simulink model "VCU_CS75_9_30"  (R2014a)
settings: Solver=FixedStepDiscrete  StartTime=0.0  StopTime=25  FixedStep=0.0005  RelTol=1e-3
undefined symbols (not defined in the file or in its folder): APAStatus_2D4, ecucoder_acal, I_SW01_L, LDW, ST_comd, TX2D4
libraries: simulink x881, ec5744lib x37
(part 29 of 30)

== system VCU_CS75_9_30/长安CS75底盘程序，20ms一次/BSW_Input/CAN1_Rx/SAS_108/ReceiveMessages/Subsystem/SAS_2 ==
  input : Inport
  Data Type Conversion : DataTypeConversion
  Demux : Demux  Outputs=8
  SAS_CRCCheck_Ad : Sum
  SAS_CRCCheck_Convert : DataTypeConversion  OutDataTypeStr=uint32
  SAS_CRCCheck_F : Gain
  SAS_CRCCheck_L : simulink/Logic and Bit Operations/Bitwise Operator  logicop=AND  UseBitMask=on  BitMask=255  BitMaskRealWorld=Stored Integer
  SAS_CRCCheck_O : Constant  Value=0  OutDataTypeStr=single
  SAS_CRCCheck_S : ArithShift
  SAS_CRCCheck_Sub : Subsystem
  SAS_CRCCheck_sat : Saturate  UpperLimit=255  LowerLimit=0
  SAS_CRCCheckcv : DataTypeConversion
  SAS_Calibrated_Ad : Sum
  SAS_Calibrated_Convert : DataTypeConversion  OutDataTypeStr=uint32
  SAS_Calibrated_F : Gain
  SAS_Calibrated_L : simulink/Logic and Bit Operations/Bitwise Operator  logicop=AND  UseBitMask=on  BitMask=32  BitMaskRealWorld=Stored Integer
  SAS_Calibrated_O : Constant  Value=0  OutDataTypeStr=single
  SAS_Calibrated_S : ArithShift  BitShiftNumber=5
  SAS_Calibrated_Sub : Subsystem
  SAS_Calibrated_sat : Saturate  UpperLimit=1  LowerLimit=0
  SAS_Calibratedcv : DataTypeConversion
  SAS_RollingCounter_Ad : Sum
  SAS_RollingCounter_Convert : DataTypeConversion  OutDataTypeStr=uint32
  SAS_RollingCounter_F : Gain
  SAS_RollingCounter_L : simulink/Logic and Bit Operations/Bitwise Operator  logicop=AND  UseBitMask=on  BitMask=15  BitMaskRealWorld=Stored Integer
  SAS_RollingCounter_O : Constant  Value=0  OutDataTypeStr=single
  SAS_RollingCounter_S : ArithShift
  SAS_RollingCounter_Sub : Subsystem
  SAS_RollingCounter_sat : Saturate  UpperLimit=15  LowerLimit=0
  SAS_RollingCountercv : DataTypeConversion
  SAS_SASFailure_Ad : Sum
  SAS_SASFailure_Convert : DataTypeConversion  OutDataTypeStr=uint32
  SAS_SASFailure_F : Gain
  SAS_SASFailure_L : simulink/Logic and Bit Operations/Bitwise Operator  logicop=AND  UseBitMask=on  BitMask=64  BitMaskRealWorld=Stored Integer
  SAS_SASFailure_O : Constant  Value=0  OutDataTypeStr=single
  SAS_SASFailure_S : ArithShift  BitShiftNumber=6
  SAS_SASFailure_Sub : Subsystem
  SAS_SASFailure_sat : Saturate  UpperLimit=1  LowerLimit=0
  SAS_SASFailurecv : DataTypeConversion
  SAS_SteeringAngleCS : ArithShift  BitShiftNumber=-16
  SAS_SteeringAngleCS1 : ArithShift  BitShiftNumber=-15
  SAS_SteeringAngleConS : Constant  OutDataTypeStr=single
  SAS_SteeringAngleMinus : UnaryMinus
  SAS_SteeringAngleROP : RelationalOperator  OutDataTypeStr=boolean
  SAS_SteeringAngleSW : Switch  Criteria=u2 ~= 0
  SAS_SteeringAngleSpeed_Ad : Sum
  SAS_SteeringAngleSpeed_Convert : DataTypeConversion  OutDataTypeStr=uint32
  SAS_SteeringAngleSpeed_F : Gain  Gain=4
  SAS_SteeringAngleSpeed_L : simulink/Logic and Bit Operations/Bitwise Operator  logicop=AND  UseBitMask=on  BitMask=255  BitMaskRealWorld=Stored Integer
  SAS_SteeringAngleSpeed_O : Constant  Value=0  OutDataTypeStr=single
  SAS_SteeringAngleSpeed_S : ArithShift
  SAS_SteeringAngleSpeed_Sub : Subsystem
  SAS_SteeringAngleSpeed_sat : Saturate  UpperLimit=1020  LowerLimit=0
  SAS_SteeringAngleSpeedcv : DataTypeConversion
  SAS_SteeringAngleValid_Ad : Sum
  SAS_SteeringAngleValid_Convert : DataTypeConversion  OutDataTypeStr=uint32
  SAS_SteeringAngleValid_F : Gain
  SAS_SteeringAngleValid_L : simulink/Logic and Bit Operations/Bitwise Operator  logicop=AND  UseBitMask=on  BitMask=128  BitMaskRealWorld=Stored Integer
  SAS_SteeringAngleValid_O : Constant  Value=0  OutDataTypeStr=single
  SAS_SteeringAngleValid_S : ArithShift  BitShiftNumber=7
  SAS_SteeringAngleValid_Sub : Subsystem
  SAS_SteeringAngleValid_sat : Saturate  UpperLimit=1  LowerLimit=0
  SAS_SteeringAngleValidcv : DataTypeConversion
  SAS_SteeringAngle_Ad : Sum
  SAS_SteeringAngle_Convert : DataTypeConversion  OutDataTypeStr=uint32
  SAS_SteeringAngle_F : Gain  Gain=0.1
  SAS_SteeringAngle_L : simulink/Logic and Bit Operations/Bitwise Operator  logicop=AND  UseBitMask=on  BitMask=65535  BitMaskRealWorld=Stored Integer
  SAS_SteeringAngle_O : Constant  Value=0  OutDataTypeStr=single
  SAS_SteeringAngle_S : ArithShift
  SAS_SteeringAngle_Sub : Subsystem
  SAS_SteeringAngle_sat : Saturate  UpperLimit=780  LowerLimit=-780
  SAS_SteeringAnglecv : DataTypeConversion
  SAS_SteeringAngleinput1_Ad : Sum
  SAS_SteeringAngleinput1_C : Constant  Value=256
  SAS_SteeringAngleinput1_P : Product
  SAS_SteeringAnglesubcon : Sum  Inputs=+-
  SAS_SteeringAngle_Out : Outport
  SAS_SteeringAngleSpeed_Out : Outport  Port=2
  SAS_Calibrated_Out : Outport  Port=3
  SAS_SASFailure_Out : Outport  Port=4
  SAS_SteeringAngleValid_Out : Outport  Port=5
  SAS_RollingCounter_Out : Outport  Port=6
  SAS_CRCCheck_Out : Outport  Port=7
  wires:
  SAS_SteeringAngle_F/1 -> SAS_SteeringAngle_Ad/1
  SAS_SteeringAngle_O/1 -> SAS_SteeringAngle_Ad/2
  SAS_SteeringAngle_Ad/1 -> SAS_SteeringAngle_sat/1
  SAS_SteeringAngle_sat/1 -> SAS_SteeringAngle_Out/1
  Demux/1 -> SAS_SteeringAngleinput1_P/1
  SAS_SteeringAngleinput1_C/1 -> SAS_SteeringAngleinput1_P/2
  SAS_SteeringAngleinput1_P/1 -> SAS_SteeringAngleinput1_Ad/1
  Demux/2 -> SAS_SteeringAngleinput1_Ad/2
  SAS_SteeringAngleinput1_Ad/1 -> SAS_SteeringAngle_Sub/1(In1)
  SAS_SteeringAngle_Sub/1(Out1) -> SAS_SteeringAngle_Convert/1
  SAS_SteeringAngle_Convert/1 -> SAS_SteeringAngle_L/1
  SAS_SteeringAngle_L/1 -> SAS_SteeringAngle_S/1
  SAS_SteeringAngle_S/1 -> SAS_SteeringAnglecv/1
  SAS_SteeringAnglecv/1 -> SAS_SteeringAngleROP/1, SAS_SteeringAnglesubcon/2, SAS_SteeringAngleSW/3
  SAS_SteeringAngleConS/1 -> SAS_SteeringAngleCS/1, SAS_SteeringAngleCS1/1
  SAS_SteeringAngleCS1/1 -> SAS_SteeringAngleROP/2
  SAS_SteeringAngleCS/1 -> SAS_SteeringAnglesubcon/1
  SAS_SteeringAnglesubcon/1 -> SAS_SteeringAngleMinus/1
  SAS_SteeringAngleMinus/1 -> SAS_SteeringAngleSW/1
  SAS_SteeringAngleSW/1 -> Data Type Conversion/1
  SAS_SteeringAngleROP/1 -> SAS_SteeringAngleSW/2
  SAS_SteeringAngleSpeed_F/1 -> SAS_SteeringAngleSpeed_Ad/1
  SAS_SteeringAngleSpeed_O/1 -> SAS_SteeringAngleSpeed_Ad/2
  SAS_SteeringAngleSpeed_Ad/1 -> SAS_SteeringAngleSpeed_sat/1
  SAS_SteeringAngleSpeed_sat/1 -> SAS_SteeringAngleSpeed_Out/1
  Demux/3 -> SAS_SteeringAngleSpeed_Sub/1(In1)
  SAS_SteeringAngleSpeed_Sub/1(Out1) -> SAS_SteeringAngleSpeed_Convert/1
  SAS_SteeringAngleSpeed_Convert/1 -> SAS_SteeringAngleSpeed_L/1
  SAS_SteeringAngleSpeed_L/1 -> SAS_SteeringAngleSpeed_S/1
  SAS_SteeringAngleSpeed_S/1 -> SAS_SteeringAngleSpeedcv/1
  SAS_SteeringAngleSpeedcv/1 -> SAS_SteeringAngleSpeed_F/1
  SAS_Calibrated_F/1 -> SAS_Calibrated_Ad/1
  SAS_Calibrated_O/1 -> SAS_Calibrated_Ad/2
  SAS_Calibrated_Ad/1 -> SAS_Calibrated_sat/1
  SAS_Calibrated_sat/1 -> SAS_Calibrated_Out/1
  Demux/4 -> SAS_Calibrated_Sub/1(In1), SAS_SASFailure_Sub/1(In1), SAS_SteeringAngleValid_Sub/1(In1)
  SAS_Calibrated_Sub/1(Out1) -> SAS_Calibrated_Convert/1
  SAS_Calibrated_Convert/1 -> SAS_Calibrated_L/1
  SAS_Calibrated_L/1 -> SAS_Calibrated_S/1
  SAS_Calibrated_S/1 -> SAS_Calibratedcv/1
  SAS_Calibratedcv/1 -> SAS_Calibrated_F/1
  SAS_SASFailure_F/1 -> SAS_SASFailure_Ad/1
  SAS_SASFailure_O/1 -> SAS_SASFailure_Ad/2
  SAS_SASFailure_Ad/1 -> SAS_SASFailure_sat/1
  SAS_SASFailure_sat/1 -> SAS_SASFailure_Out/1
  SAS_SASFailure_Sub/1(Out1) -> SAS_SASFailure_Convert/1
  SAS_SASFailure_Convert/1 -> SAS_SASFailure_L/1
  SAS_SASFailure_L/1 -> SAS_SASFailure_S/1
  SAS_SASFailure_S/1 -> SAS_SASFailurecv/1
  SAS_SASFailurecv/1 -> SAS_SASFailure_F/1
  SAS_SteeringAngleValid_F/1 -> SAS_SteeringAngleValid_Ad/1
  SAS_SteeringAngleValid_O/1 -> SAS_SteeringAngleValid_Ad/2
  SAS_SteeringAngleValid_Ad/1 -> SAS_SteeringAngleValid_sat/1
  SAS_SteeringAngleValid_sat/1 -> SAS_SteeringAngleValid_Out/1
  SAS_SteeringAngleValid_Sub/1(Out1) -> SAS_SteeringAngleValid_Convert/1
  SAS_SteeringAngleValid_Convert/1 -> SAS_SteeringAngleValid_L/1
  SAS_SteeringAngleValid_L/1 -> SAS_SteeringAngleValid_S/1
  SAS_SteeringAngleValid_S/1 -> SAS_SteeringAngleValidcv/1
  SAS_SteeringAngleValidcv/1 -> SAS_SteeringAngleValid_F/1
  SAS_RollingCounter_F/1 -> SAS_RollingCounter_Ad/1
  SAS_RollingCounter_O/1 -> SAS_RollingCounter_Ad/2
  SAS_RollingCounter_Ad/1 -> SAS_RollingCounter_sat/1
  SAS_RollingCounter_sat/1 -> SAS_RollingCounter_Out/1
  Demux/7 -> SAS_RollingCounter_Sub/1(In1)
  SAS_RollingCounter_Sub/1(Out1) -> SAS_RollingCounter_Convert/1
  SAS_RollingCounter_Convert/1 -> SAS_RollingCounter_L/1
  SAS_RollingCounter_L/1 -> SAS_RollingCounter_S/1
  SAS_RollingCounter_S/1 -> SAS_RollingCountercv/1
  SAS_RollingCountercv/1 -> SAS_RollingCounter_F/1
  SAS_CRCCheck_F/1 -> SAS_CRCCheck_Ad/1
  SAS_CRCCheck_O/1 -> SAS_CRCCheck_Ad/2
  SAS_CRCCheck_Ad/1 -> SAS_CRCCheck_sat/1
  SAS_CRCCheck_sat/1 -> SAS_CRCCheck_Out/1
  Demux/8 -> SAS_CRCCheck_Sub/1(In1)
  SAS_CRCCheck_Sub/1(Out1) -> SAS_CRCCheck_Convert/1
  SAS_CRCCheck_Convert/1 -> SAS_CRCCheck_L/1
  SAS_CRCCheck_L/1 -> SAS_CRCCheck_S/1
  SAS_CRCCheck_S/1 -> SAS_CRCCheckcv/1
  SAS_CRCCheckcv/1 -> SAS_CRCCheck_F/1
  input/1 -> Demux/1
  Data Type Conversion/1 -> SAS_SteeringAngle_F/1

== system VCU_CS75_9_30/长安CS75底盘程序，20ms一次/BSW_Input/CAN1_Rx/SCM_3B8/ReceiveMessages/Subsystem/SCM_3B2 ==
  input : Inport
  Demux : Demux  Outputs=8
  SCM_ACCCancel_Ad : Sum
  SCM_ACCCancel_Convert : DataTypeConversion  OutDataTypeStr=uint32
  SCM_ACCCancel_F : Gain
  SCM_ACCCancel_L : simulink/Logic and Bit Operations/Bitwise Operator  logicop=AND  UseBitMask=on  BitMask=4  BitMaskRealWorld=Stored Integer
  SCM_ACCCancel_O : Constant  Value=0  OutDataTypeStr=single
  SCM_ACCCancel_S : ArithShift  BitShiftNumber=2
  SCM_ACCCancel_Sub : Subsystem
  SCM_ACCCancel_sat : Saturate  UpperLimit=0  LowerLimit=0
  SCM_ACCCancelcv : DataTypeConversion
  SCM_ACCOn_Ad : Sum
  SCM_ACCOn_Convert : DataTypeConversion  OutDataTypeStr=uint32
  SCM_ACCOn_F : Gain
  SCM_ACCOn_L : simulink/Logic and Bit Operations/Bitwise Operator  logicop=AND  UseBitMask=on  BitMask=1  BitMaskRealWorld=Stored Integer
  SCM_ACCOn_O : Constant  Value=0  OutDataTypeStr=single
  SCM_ACCOn_S : ArithShift
  SCM_ACCOn_Sub : Subsystem
  SCM_ACCOn_sat : Saturate  UpperLimit=0  LowerLimit=0
  SCM_ACCOncv : DataTypeConversion
  SCM_IACCOn_Ad : Sum
  SCM_IACCOn_Convert : DataTypeConversion  OutDataTypeStr=uint32
  SCM_IACCOn_F : Gain
  SCM_IACCOn_L : simulink/Logic and Bit Operations/Bitwise Operator  logicop=AND  UseBitMask=on  BitMask=16  BitMaskRealWorld=Stored Integer
  SCM_IACCOn_O : Constant  Value=0  OutDataTypeStr=single
  SCM_IACCOn_S : ArithShift  BitShiftNumber=4
  SCM_IACCOn_Sub : Subsystem
  SCM_IACCOn_sat : Saturate  UpperLimit=0  LowerLimit=0
  SCM_IACCOncv : DataTypeConversion
  SCM_Resume_Ad : Sum
  SCM_Resume_Convert : DataTypeConversion  OutDataTypeStr=uint32
  SCM_Resume_F : Gain
  SCM_Resume_L : simulink/Logic and Bit Operations/Bitwise Operator  logicop=AND  UseBitMask=on  BitMask=16  BitMaskRealWorld=Stored Integer
  SCM_Resume_O : Constant  Value=0  OutDataTypeStr=single
  SCM_Resume_S : ArithShift  BitShiftNumber=4
  SCM_Resume_Sub : Subsystem
  SCM_Resume_sat : Saturate  UpperLimit=0  LowerLimit=0
  SCM_Resumecv : DataTypeConversion
  SCM_Speeddecrease_Ad : Sum
  SCM_Speeddecrease_Convert : DataTypeConversion  OutDataTypeStr=uint32
  SCM_Speeddecrease_F : Gain
  SCM_Speeddecrease_L : simulink/Logic and Bit Operations/Bitwise Operator  logicop=AND  UseBitMask=on  BitMask=64  BitMaskRealWorld=Stored Integer
  SCM_Speeddecrease_O : Constant  Value=0  OutDataTypeStr=single
  SCM_Speeddecrease_S : ArithShift  BitShiftNumber=6
  SCM_Speeddecrease_Sub : Subsystem
  SCM_Speeddecrease_sat : Saturate  UpperLimit=0  LowerLimit=0
  SCM_Speeddecreasecv : DataTypeConversion
  SCM_TimeGap_Ad : Sum
  SCM_TimeGap_Convert : DataTypeConversion  OutDataTypeStr=uint32
  SCM_TimeGap_F : Gain
  SCM_TimeGap_L : simulink/Logic and Bit Operations/Bitwise Operator  logicop=AND  UseBitMask=on  BitMask=1  BitMaskRealWorld=Stored Integer
  SCM_TimeGap_O : Constant  Value=0  OutDataTypeStr=single
  SCM_TimeGap_S : ArithShift
  SCM_TimeGap_Sub : Subsystem
  SCM_TimeGap_sat : Saturate  UpperLimit=0  LowerLimit=0
  SCM_TimeGapcv : DataTypeConversion
  SCM_ACCOn_Out : Outport
  SCM_ACCCancel_Out : Outport  Port=2
  SCM_Resume_Out : Outport  Port=3
  SCM_Speeddecrease_Out : Outport  Port=4
  SCM_TimeGap_Out : Outport  Port=5
  SCM_IACCOn_Out : Outport  Port=6
  wires:
  SCM_ACCOn_F/1 -> SCM_ACCOn_Ad/1
  SCM_ACCOn_O/1 -> SCM_ACCOn_Ad/2
  SCM_ACCOn_Ad/1 -> SCM_ACCOn_sat/1
  SCM_ACCOn_sat/1 -> SCM_ACCOn_Out/1
  Demux/1 -> SCM_ACCOn_Sub/1(In1), SCM_ACCCancel_Sub/1(In1), SCM_Resume_Sub/1(In1), SCM_Speeddecrease_Sub/1(In1)
  SCM_ACCOn_Sub/1(Out1) -> SCM_ACCOn_Convert/1
  SCM_ACCOn_Convert/1 -> SCM_ACCOn_L/1
  SCM_ACCOn_L/1 -> SCM_ACCOn_S/1
  SCM_ACCOn_S/1 -> SCM_ACCOncv/1
  SCM_ACCOncv/1 -> SCM_ACCOn_F/1
  SCM_ACCCancel_F/1 -> SCM_ACCCancel_Ad/1
  SCM_ACCCancel_O/1 -> SCM_ACCCancel_Ad/2
  SCM_ACCCancel_Ad/1 -> SCM_ACCCancel_sat/1
  SCM_ACCCancel_sat/1 -> SCM_ACCCancel_Out/1
  SCM_ACCCancel_Sub/1(Out1) -> SCM_ACCCancel_Convert/1
  SCM_ACCCancel_Convert/1 -> SCM_ACCCancel_L/1
  SCM_ACCCancel_L/1 -> SCM_ACCCancel_S/1
  SCM_ACCCancel_S/1 -> SCM_ACCCancelcv/1
  SCM_ACCCancelcv/1 -> SCM_ACCCancel_F/1
  SCM_Resume_F/1 -> SCM_Resume_Ad/1
  SCM_Resume_O/1 -> SCM_Resume_Ad/2
  SCM_Resume_Ad/1 -> SCM_Resume_sat/1
  SCM_Resume_sat/1 -> SCM_Resume_Out/1
  SCM_Resume_Sub/1(Out1) -> SCM_Resume_Convert/1
  SCM_Resume_Convert/1 -> SCM_Resume_L/1
  SCM_Resume_L/1 -> SCM_Resume_S/1
  SCM_Resume_S/1 -> SCM_Resumecv/1
  SCM_Resumecv/1 -> SCM_Resume_F/1
  SCM_Speeddecrease_F/1 -> SCM_Speeddecrease_Ad/1
  SCM_Speeddecrease_O/1 -> SCM_Speeddecrease_Ad/2
  SCM_Speeddecrease_Ad/1 -> SCM_Speeddecrease_sat/1
  SCM_Speeddecrease_sat/1 -> SCM_Speeddecrease_Out/1
  SCM_Speeddecrease_Sub/1(Out1) -> SCM_Speeddecrease_Convert/1
  SCM_Speeddecrease_Convert/1 -> SCM_Speeddecrease_L/1
  SCM_Speeddecrease_L/1 -> SCM_Speeddecrease_S/1
  SCM_Speeddecrease_S/1 -> SCM_Speeddecreasecv/1
  SCM_Speeddecreasecv/1 -> SCM_Speeddecrease_F/1
  SCM_TimeGap_F/1 -> SCM_TimeGap_Ad/1
  SCM_TimeGap_O/1 -> SCM_TimeGap_Ad/2
  SCM_TimeGap_Ad/1 -> SCM_TimeGap_sat/1
  SCM_TimeGap_sat/1 -> SCM_TimeGap_Out/1
  Demux/2 -> SCM_TimeGap_Sub/1(In1), SCM_IACCOn_Sub/1(In1)
  SCM_TimeGap_Sub/1(Out1) -> SCM_TimeGap_Convert/1
  SCM_TimeGap_Convert/1 -> SCM_TimeGap_L/1
  SCM_TimeGap_L/1 -> SCM_TimeGap_S/1
  SCM_TimeGap_S/1 -> SCM_TimeGapcv/1
  SCM_TimeGapcv/1 -> SCM_TimeGap_F/1
  SCM_IACCOn_F/1 -> SCM_IACCOn_Ad/1
  SCM_IACCOn_O/1 -> SCM_IACCOn_Ad/2
  SCM_IACCOn_Ad/1 -> SCM_IACCOn_sat/1
  SCM_IACCOn_sat/1 -> SCM_IACCOn_Out/1
  SCM_IACCOn_Sub/1(Out1) -> SCM_IACCOn_Convert/1
  SCM_IACCOn_Convert/1 -> SCM_IACCOn_L/1
  SCM_IACCOn_L/1 -> SCM_IACCOn_S/1
  SCM_IACCOn_S/1 -> SCM_IACCOncv/1
  SCM_IACCOncv/1 -> SCM_IACCOn_F/1
  input/1 -> Demux/1

== system VCU_CS75_9_30/长安CS75底盘程序，20ms一次/BSW_Input/CAN1_Rx/SRS_005/ReceiveMessages/Subsystem/SRS_1 ==
  input : Inport
  Demux : Demux  Outputs=8
  SRS_DriverBuckleSwitchStatus_Ad : Sum
  SRS_DriverBuckleSwitchStatus_Convert : DataTypeConversion  OutDataTypeStr=uint32
  SRS_DriverBuckleSwitchStatus_F : Gain
  SRS_DriverBuckleSwitchStatus_L : simulink/Logic and Bit Operations/Bitwise Operator  logicop=AND  UseBitMask=on  BitMask=192  BitMaskRealWorld=Stored Integer
  SRS_DriverBuckleSwitchStatus_O : Constant  Value=0  OutDataTypeStr=single
  SRS_DriverBuckleSwitchStatus_S : ArithShift  BitShiftNumber=6
  SRS_DriverBuckleSwitchStatus_Sub : Subsystem
  SRS_DriverBuckleSwitchStatus_sat : Saturate  UpperLimit=3  LowerLimit=0
  SRS_DriverBuckleSwitchStatuscv : DataTypeConversion
  SRS_RollingCounter_Ad : Sum
  SRS_RollingCounter_Convert : DataTypeConversion  OutDataTypeStr=uint32
  SRS_RollingCounter_F : Gain
  SRS_RollingCounter_L : simulink/Logic and Bit Operations/Bitwise Operator  logicop=AND  UseBitMask=on  BitMask=15  BitMaskRealWorld=Stored Integer
  SRS_RollingCounter_O : Constant  Value=0  OutDataTypeStr=single
  SRS_RollingCounter_S : ArithShift
  SRS_RollingCounter_Sub : Subsystem
  SRS_RollingCounter_sat : Saturate  UpperLimit=15  LowerLimit=0
  SRS_RollingCountercv : DataTypeConversion
  SRS_DriverBuckleSwitchStatus_Out : Outport
  SRS_RollingCounter_Out : Outport  Port=2
  wires:
  input/1 -> Demux/1
  SRS_RollingCountercv/1 -> SRS_RollingCounter_F/1
  SRS_RollingCounter_S/1 -> SRS_RollingCountercv/1
  SRS_RollingCounter_L/1 -> SRS_RollingCounter_S/1
  SRS_RollingCounter_Convert/1 -> SRS_RollingCounter_L/1
  SRS_RollingCounter_Sub/1(Out1) -> SRS_RollingCounter_Convert/1
  Demux/4 -> SRS_RollingCounter_Sub/1(In1)
  SRS_RollingCounter_sat/1 -> SRS_RollingCounter_Out/1
  SRS_RollingCounter_Ad/1 -> SRS_RollingCounter_sat/1
  SRS_RollingCounter_O/1 -> SRS_RollingCounter_Ad/2
  SRS_RollingCounter_F/1 -> SRS_RollingCounter_Ad/1
  SRS_DriverBuckleSwitchStatuscv/1 -> SRS_DriverBuckleSwitchStatus_F/1
  SRS_DriverBuckleSwitchStatus_S/1 -> SRS_DriverBuckleSwitchStatuscv/1
  SRS_DriverBuckleSwitchStatus_L/1 -> SRS_DriverBuckleSwitchStatus_S/1
  SRS_DriverBuckleSwitchStatus_Convert/1 -> SRS_DriverBuckleSwitchStatus_L/1
  SRS_DriverBuckleSwitchStatus_Sub/1(Out1) -> SRS_DriverBuckleSwitchStatus_Convert/1
  Demux/2 -> SRS_DriverBuckleSwitchStatus_Sub/1(In1)
  SRS_DriverBuckleSwitchStatus_sat/1 -> SRS_DriverBuckleSwitchStatus_Out/1
  SRS_DriverBuckleSwitchStatus_Ad/1 -> SRS_DriverBuckleSwitchStatus_sat/1
  SRS_DriverBuckleSwitchStatus_O/1 -> SRS_DriverBuckleSwitchStatus_Ad/2
  SRS_DriverBuckleSwitchStatus_F/1 -> SRS_DriverBuckleSwitchStatus_Ad/1

== system VCU_CS75_9_30/长安CS75底盘程序，20ms一次/BSW_Input/CAN1_Rx/TCU_286/ReceiveMessages/Subsystem/TCU_1 ==
  input : Inport
  Demux : Demux  Outputs=8
  TCU_ActualGearValid_Ad : Sum
  TCU_ActualGearValid_Convert : DataTypeConversion  OutDataTypeStr=uint32
  TCU_ActualGearValid_F : Gain
  TCU_ActualGearValid_L : simulink/Logic and Bit Operations/Bitwise Operator  logicop=AND  UseBitMask=on  BitMask=32  BitMaskRealWorld=Stored Integer
  TCU_ActualGearValid_O : Constant  Value=0  OutDataTypeStr=single
  TCU_ActualGearValid_S : ArithShift  BitShiftNumber=5
  TCU_ActualGearValid_Sub : Subsystem
  TCU_ActualGearValid_sat : Saturate  UpperLimit=1  LowerLimit=0
  TCU_ActualGearValidcv : DataTypeConversion
  TCU_ActualGear_Ad : Sum
  TCU_ActualGear_Convert : DataTypeConversion  OutDataTypeStr=uint32
  TCU_ActualGear_F : Gain
  TCU_ActualGear_L : simulink/Logic and Bit Operations/Bitwise Operator  logicop=AND  UseBitMask=on  BitMask=15  BitMaskRealWorld=Stored Integer
  TCU_ActualGear_O : Constant  Value=0  OutDataTypeStr=single
  TCU_ActualGear_S : ArithShift
  TCU_ActualGear_Sub : Subsystem
  TCU_ActualGear_sat : Saturate  UpperLimit=15  LowerLimit=0
  TCU_ActualGearcv : DataTypeConversion
  TCU_GearShiftPosition_Ad : Sum
  TCU_GearShiftPosition_Convert : DataTypeConversion  OutDataTypeStr=uint32
  TCU_GearShiftPosition_F : Gain
  TCU_GearShiftPosition_L : simulink/Logic and Bit Operations/Bitwise Operator  logicop=AND  UseBitMask=on  BitMask=240  BitMaskRealWorld=Stored Integer
  TCU_GearShiftPosition_O : Constant  Value=0  OutDataTypeStr=single
  TCU_GearShiftPosition_S : ArithShift  BitShiftNumber=4
  TCU_GearShiftPosition_Sub : Subsystem
  TCU_GearShiftPosition_sat : Saturate  UpperLimit=15  LowerLimit=0
  TCU_GearShiftPositioncv : DataTypeConversion
  TCU_ShiftPositionValid_Ad : Sum
  TCU_ShiftPositionValid_Convert : DataTypeConversion  OutDataTypeStr=uint32
  TCU_ShiftPositionValid_F : Gain
  TCU_ShiftPositionValid_L : simulink/Logic and Bit Operations/Bitwise Operator  logicop=AND  UseBitMask=on  BitMask=16  BitMaskRealWorld=Stored Integer
  TCU_ShiftPositionValid_O : Constant  Value=0  OutDataTypeStr=single
  TCU_ShiftPositionValid_S : ArithShift  BitShiftNumber=4
  TCU_ShiftPositionValid_Sub : Subsystem
  TCU_ShiftPositionValid_sat : Saturate  UpperLimit=1  LowerLimit=0
  TCU_ShiftPositionValidcv : DataTypeConversion
  TCU_ActualGear_Out : Outport
  TCU_ShiftPositionValid_Out : Outport  Port=2
  TCU_ActualGearValid_Out : Outport  Port=3
  TCU_GearShiftPosition_Out : Outport  Port=4
  wires:
  input/1 -> Demux/1
  TCU_GearShiftPositioncv/1 -> TCU_GearShiftPosition_F/1
  TCU_GearShiftPosition_S/1 -> TCU_GearShiftPositioncv/1
  TCU_GearShiftPosition_L/1 -> TCU_GearShiftPosition_S/1
  TCU_GearShiftPosition_Convert/1 -> TCU_GearShiftPosition_L/1
  TCU_GearShiftPosition_Sub/1(Out1) -> TCU_GearShiftPosition_Convert/1
  Demux/3 -> TCU_GearShiftPosition_Sub/1(In1)
  TCU_GearShiftPosition_sat/1 -> TCU_GearShiftPosition_Out/1
  TCU_GearShiftPosition_Ad/1 -> TCU_GearShiftPosition_sat/1
  TCU_GearShiftPosition_O/1 -> TCU_GearShiftPosition_Ad/2
  TCU_GearShiftPosition_F/1 -> TCU_GearShiftPosition_Ad/1
  TCU_ActualGearValidcv/1 -> TCU_ActualGearValid_F/1
  TCU_ActualGearValid_S/1 -> TCU_ActualGearValidcv/1
  TCU_ActualGearValid_L/1 -> TCU_ActualGearValid_S/1
  TCU_ActualGearValid_Convert/1 -> TCU_ActualGearValid_L/1
  TCU_ActualGearValid_Sub/1(Out1) -> TCU_ActualGearValid_Convert/1
  TCU_ActualGearValid_sat/1 -> TCU_ActualGearValid_Out/1
  TCU_ActualGearValid_Ad/1 -> TCU_ActualGearValid_sat/1
  TCU_ActualGearValid_O/1 -> TCU_ActualGearValid_Ad/2
  TCU_ActualGearValid_F/1 -> TCU_ActualGearValid_Ad/1
  TCU_ShiftPositionValidcv/1 -> TCU_ShiftPositionValid_F/1
  TCU_ShiftPositionValid_S/1 -> TCU_ShiftPositionValidcv/1
  TCU_ShiftPositionValid_L/1 -> TCU_ShiftPositionValid_S/1
  TCU_ShiftPositionValid_Convert/1 -> TCU_ShiftPositionValid_L/1
  TCU_ShiftPositionValid_Sub/1(Out1) -> TCU_ShiftPositionValid_Convert/1
  TCU_ShiftPositionValid_sat/1 -> TCU_ShiftPositionValid_Out/1
  TCU_ShiftPositionValid_Ad/1 -> TCU_ShiftPositionValid_sat/1
  TCU_ShiftPositionValid_O/1 -> TCU_ShiftPositionValid_Ad/2
  TCU_ShiftPositionValid_F/1 -> TCU_ShiftPositionValid_Ad/1
  TCU_ActualGearcv/1 -> TCU_ActualGear_F/1
  TCU_ActualGear_S/1 -> TCU_ActualGearcv/1
  TCU_ActualGear_L/1 -> TCU_ActualGear_S/1
  TCU_ActualGear_Convert/1 -> TCU_ActualGear_L/1
  TCU_ActualGear_Sub/1(Out1) -> TCU_ActualGear_Convert/1
  Demux/2 -> TCU_ActualGearValid_Sub/1(In1), TCU_ShiftPositionValid_Sub/1(In1), TCU_ActualGear_Sub/1(In1)
  TCU_ActualGear_sat/1 -> TCU_ActualGear_Out/1
  TCU_ActualGear_Ad/1 -> TCU_ActualGear_sat/1
  TCU_ActualGear_O/1 -> TCU_ActualGear_Ad/2
  TCU_ActualGear_F/1 -> TCU_ActualGear_Ad/1

== system VCU_CS75_9_30/长安CS75底盘程序，20ms一次/BSW_Output/CAN1_Tx/Subsystem/to28A/APA_28A1/APA_CheckSum ==
  APA_CheckSum : Inport
  APA_CheckSumRon : Rounding  Operator=round
  APA_CheckSum_1sat : Saturate  UpperLimit=255  LowerLimit=0
  APA_CheckSum_Convert : DataTypeConversion  OutDataTypeStr=uint8
  APA_CheckSum_Convert1 : DataTypeConversion  OutDataTypeStr=uint32
  APA_CheckSum_D : Product  Inputs=*/
  APA_CheckSum_F : Constant  OutDataTypeStr=single
  APA_CheckSum_L : simulink/Logic and Bit Operations/Bitwise Operator  logicop=AND  UseBitMask=on  BitMask=255  BitMaskRealWorld=Stored Integer
  APA_CheckSum_O : Constant  Value=0  OutDataTypeStr=single
  APA_CheckSum_S : ArithShift
  APA_CheckSum_sat : Saturate  UpperLimit=255  LowerLimit=0
  APA_CheckSum_st : Sum  Inputs=+-
  Constant{1..7} (7 alike) : Constant  Value=0  OutDataTypeStr=uint8
  output1 : Outport
  output2 : Outport  Port=2
  output3 : Outport  Port=3
  output4 : Outport  Port=4
  output5 : Outport  Port=5
  output6 : Outport  Port=6
  output7 : Outport  Port=7
  output8 : Outport  Port=8
  wires:
  APA_CheckSum/1 -> APA_CheckSum_sat/1
  APA_CheckSum_sat/1 -> APA_CheckSum_st/1
  APA_CheckSum_O/1 -> APA_CheckSum_st/2
  APA_CheckSum_st/1 -> APA_CheckSum_D/1
  APA_CheckSum_F/1 -> APA_CheckSum_D/2
  APA_CheckSum_D/1 -> APA_CheckSumRon/1
  APA_CheckSumRon/1 -> APA_CheckSum_S/1
  APA_CheckSum_S/1 -> APA_CheckSum_1sat/1
  APA_CheckSum_1sat/1 -> APA_CheckSum_Convert1/1
  APA_CheckSum_Convert1/1 -> APA_CheckSum_L/1
  APA_CheckSum_L/1 -> APA_CheckSum_Convert/1
  APA_CheckSum_Convert/1 -> output8/1
  Constant1/1 -> output1/1
  Constant2/1 -> output2/1
  Constant3/1 -> output3/1
  Constant4/1 -> output4/1
  Constant5/1 -> output5/1
  Constant6/1 -> output6/1
  Constant7/1 -> output7/1

== system VCU_CS75_9_30/长安CS75底盘程序，20ms一次/BSW_Output/CAN1_Tx/Subsystem/to28A/APA_28A1/APA_EPSAngleReq ==
  APA_EPSAngleReq : Inport
  APA_EPSAngleReqABS : Abs
  APA_EPSAngleReqBitCov : DataTypeConversion  OutDataTypeStr=uint32
  APA_EPSAngleReqBitCov1 : DataTypeConversion  OutDataTypeStr=uint8
  APA_EPSAngleReqCOV : DataTypeConversion  OutDataTypeStr=uint8
  APA_EPSAngleReqCOV1 : DataTypeConversion  OutDataTypeStr=uint8
  APA_EPSAngleReqCS : ArithShift  BitShiftNumber=-16
  APA_EPSAngleReqConS : Constant  OutDataTypeStr=single
  APA_EPSAngleReqCosR : Constant  Value=0  OutDataTypeStr=uint8
  APA_EPSAngleReqROP : RelationalOperator  Operator=<  OutDataTypeStr=boolean
  APA_EPSAngleReqRon : Rounding  Operator=round
  APA_EPSAngleReqSW : Switch  Criteria=u2 ~= 0
  APA_EPSAngleReq_1sat : Saturate  UpperLimit=1048560  LowerLimit=0
  APA_EPSAngleReq_And : simulink/Logic and Bit Operations/Bitwise Operator  logicop=AND  UseBitMask=off  NumInputPorts=2  BitMask=bin2dec('11011001')  BitMaskRealWorld=Stored Integer
  APA_EPSAngleReq_And1 : simulink/Logic and Bit Operations/Bitwise Operator  logicop=AND  UseBitMask=off  NumInputPorts=2  BitMask=bin2dec('11011001')  BitMaskRealWorld=Stored Integer
  APA_EPSAngleReq_And1_C : Constant  Value=255  OutDataTypeStr=uint32
  APA_EPSAngleReq_And_C : Constant  Value=65535
  APA_EPSAngleReq_Convert : DataTypeConversion  OutDataTypeStr=uint32
  APA_EPSAngleReq_D : Product  Inputs=*/
  APA_EPSAngleReq_D1 : Product  Inputs=*/
  APA_EPSAngleReq_D2 : Product  Inputs=*/
  APA_EPSAngleReq_F : Constant  Value=0.1  OutDataTypeStr=single
  APA_EPSAngleReq_L : simulink/Logic and Bit Operations/Bitwise Operator  logicop=AND  UseBitMask=on  BitMask=1048560  BitMaskRealWorld=Stored Integer
  APA_EPSAngleReq_O : Constant  Value=0  OutDataTypeStr=single
  APA_EPSAngleReq_S : ArithShift  BitShiftNumber=-4
  APA_EPSAngleReq_sat : Saturate  UpperLimit=3276.7  LowerLimit=-3276.8
  APA_EPSAngleReq_st : Sum  Inputs=+-
  APA_EPSAngleReqoutput2_C : Constant  Value=65536
  APA_EPSAngleReqoutput3_C : Constant  Value=256
  APA_EPSAngleReqsubcon : Sum  Inputs=+-
  Constant{1,5..8} (5 alike) : Constant  Value=0  OutDataTypeStr=uint8
  output1 : Outport
  output2 : Outport  Port=2
  output3 : Outport  Port=3
  output4 : Outport  Port=4
  output5 : Outport  Port=5
  output6 : Outport  Port=6
  output7 : Outport  Port=7
  output8 : Outport  Port=8
  wires:
  APA_EPSAngleReq/1 -> APA_EPSAngleReq_sat/1
  APA_EPSAngleReq_sat/1 -> APA_EPSAngleReq_st/1
  APA_EPSAngleReq_O/1 -> APA_EPSAngleReq_st/2
  APA_EPSAngleReq_st/1 -> APA_EPSAngleReq_D/1
  APA_EPSAngleReq_F/1 -> APA_EPSAngleReq_D/2
  APA_EPSAngleReq_D/1 -> APA_EPSAngleReqRon/1
  APA_EPSAngleReqRon/1 -> APA_EPSAngleReqROP/1, APA_EPSAngleReqABS/1, APA_EPSAngleReqSW/3
  APA_EPSAngleReqCosR/1 -> APA_EPSAngleReqROP/2
  APA_EPSAngleReqConS/1 -> APA_EPSAngleReqCS/1
  APA_EPSAngleReqCS/1 -> APA_EPSAngleReqsubcon/1
  APA_EPSAngleReqABS/1 -> APA_EPSAngleReqsubcon/2
  APA_EPSAngleReqsubcon/1 -> APA_EPSAngleReqSW/1
  APA_EPSAngleReqROP/1 -> APA_EPSAngleReqSW/2
  APA_EPSAngleReqSW/1 -> APA_EPSAngleReq_S/1
  APA_EPSAngleReq_S/1 -> APA_EPSAngleReq_1sat/1
  APA_EPSAngleReq_1sat/1 -> APA_EPSAngleReq_Convert/1
  APA_EPSAngleReq_Convert/1 -> APA_EPSAngleReq_L/1
  APA_EPSAngleReq_L/1 -> APA_EPSAngleReq_D1/1, APA_EPSAngleReq_And/1, APA_EPSAngleReq_And1/1
  APA_EPSAngleReqoutput2_C/1 -> APA_EPSAngleReq_D1/2
  APA_EPSAngleReq_D1/1 -> APA_EPSAngleReqCOV/1
  APA_EPSAngleReqCOV/1 -> output2/1
  APA_EPSAngleReq_And_C/1 -> APA_EPSAngleReqBitCov/1
  APA_EPSAngleReqBitCov/1 -> APA_EPSAngleReq_And/2
  APA_EPSAngleReq_And/1 -> APA_EPSAngleReq_D2/1
  APA_EPSAngleReqoutput3_C/1 -> APA_EPSAngleReq_D2/2
  APA_EPSAngleReq_D2/1 -> APA_EPSAngleReqCOV1/1
  APA_EPSAngleReqCOV1/1 -> output3/1
  APA_EPSAngleReq_And1_C/1 -> APA_EPSAngleReq_And1/2
  APA_EPSAngleReq_And1/1 -> APA_EPSAngleReqBitCov1/1
  APA_EPSAngleReqBitCov1/1 -> output4/1
  Constant1/1 -> output1/1
  Constant5/1 -> output5/1
  Constant6/1 -> output6/1
  Constant7/1 -> output7/1
  Constant8/1 -> output8/1

== system VCU_CS75_9_30/长安CS75底盘程序，20ms一次/BSW_Output/CAN1_Tx/Subsystem/to28A/APA_28A1/APA_IncreasePressureReq ==
  APA_IncreasePressureReq : Inport
  APA_IncreasePressureReqRon : Rounding  Operator=round
  APA_IncreasePressureReq_1sat : Saturate  UpperLimit=128  LowerLimit=0
  APA_IncreasePressureReq_Convert : DataTypeConversion  OutDataTypeStr=uint8
  APA_IncreasePressureReq_Convert1 : DataTypeConversion  OutDataTypeStr=uint32
  APA_IncreasePressureReq_D : Product  Inputs=*/
  APA_IncreasePressureReq_F : Constant  OutDataTypeStr=single
  APA_IncreasePressureReq_L : simulink/Logic and Bit Operations/Bitwise Operator  logicop=AND  UseBitMask=on  BitMask=128  BitMaskRealWorld=Stored Integer
  APA_IncreasePressureReq_O : Constant  Value=0  OutDataTypeStr=single
  APA_IncreasePressureReq_S : ArithShift  BitShiftNumber=-7
  APA_IncreasePressureReq_sat : Saturate  UpperLimit=0  LowerLimit=0
  APA_IncreasePressureReq_st : Sum  Inputs=+-
  Constant{1,3..8} (7 alike) : Constant  Value=0  OutDataTypeStr=uint8
  output1 : Outport
  output2 : Outport  Port=2
  output3 : Outport  Port=3
  output4 : Outport  Port=4
  output5 : Outport  Port=5
  output6 : Outport  Port=6
  output7 : Outport  Port=7
  output8 : Outport  Port=8
  wires:
  APA_IncreasePressureReq/1 -> APA_IncreasePressureReq_sat/1
  APA_IncreasePressureReq_sat/1 -> APA_IncreasePressureReq_st/1
  APA_IncreasePressureReq_O/1 -> APA_IncreasePressureReq_st/2
  APA_IncreasePressureReq_st/1 -> APA_IncreasePressureReq_D/1
  APA_IncreasePressureReq_F/1 -> APA_IncreasePressureReq_D/2
  APA_IncreasePressureReq_D/1 -> APA_IncreasePressureReqRon/1
  APA_IncreasePressureReqRon/1 -> APA_IncreasePressureReq_S/1
  APA_IncreasePressureReq_S/1 -> APA_IncreasePressureReq_1sat/1
  APA_IncreasePressureReq_1sat/1 -> APA_IncreasePressureReq_Convert1/1
  APA_IncreasePressureReq_Convert1/1 -> APA_IncreasePressureReq_L/1
  APA_IncreasePressureReq_L/1 -> APA_IncreasePressureReq_Convert/1
  APA_IncreasePressureReq_Convert/1 -> output2/1
  Constant1/1 -> output1/1
  Constant3/1 -> output3/1
  Constant4/1 -> output4/1
  Constant5/1 -> output5/1
  Constant6/1 -> output6/1
  Constant7/1 -> output7/1
  Constant8/1 -> output8/1

== system VCU_CS75_9_30/长安CS75底盘程序，20ms一次/BSW_Output/CAN1_Tx/Subsystem/to28A/APA_28A1/APA_Indication ==
  APA_Indication : Inport
  APA_IndicationRon : Rounding  Operator=round
  APA_Indication_1sat : Saturate  UpperLimit=56  LowerLimit=0
  APA_Indication_Convert : DataTypeConversion  OutDataTypeStr=uint8
  APA_Indication_Convert1 : DataTypeConversion  OutDataTypeStr=uint32
  APA_Indication_D : Product  Inputs=*/
  APA_Indication_F : Constant  OutDataTypeStr=single
  APA_Indication_L : simulink/Logic and Bit Operations/Bitwise Operator  logicop=AND  UseBitMask=on  BitMask=56  BitMaskRealWorld=Stored Integer
  APA_Indication_O : Constant  Value=0  OutDataTypeStr=single
  APA_Indication_S : ArithShift  BitShiftNumber=-3
  APA_Indication_sat : Saturate  UpperLimit=7  LowerLimit=0
  APA_Indication_st : Sum  Inputs=+-
  Constant{2..8} (7 alike) : Constant  Value=0  OutDataTypeStr=uint8
  output1 : Outport
  output2 : Outport  Port=2
  output3 : Outport  Port=3
  output4 : Outport  Port=4
  output5 : Outport  Port=5
  output6 : Outport  Port=6
  output7 : Outport  Port=7
  output8 : Outport  Port=8
  wires:
  APA_Indication/1 -> APA_Indication_sat/1
  APA_Indication_sat/1 -> APA_Indication_st/1
  APA_Indication_O/1 -> APA_Indication_st/2
  APA_Indication_st/1 -> APA_Indication_D/1
  APA_Indication_F/1 -> APA_Indication_D/2
  APA_Indication_D/1 -> APA_IndicationRon/1
  APA_IndicationRon/1 -> APA_Indication_S/1
  APA_Indication_S/1 -> APA_Indication_1sat/1
  APA_Indication_1sat/1 -> APA_Indication_Convert1/1
  APA_Indication_Convert1/1 -> APA_Indication_L/1
  APA_Indication_L/1 -> APA_Indication_Convert/1
  APA_Indication_Convert/1 -> output1/1
  Constant2/1 -> output2/1
  Constant3/1 -> output3/1
  Constant4/1 -> output4/1
  Constant5/1 -> output5/1
  Constant6/1 -> output6/1
  Constant7/1 -> output7/1
  Constant8/1 -> output8/1

== system VCU_CS75_9_30/长安CS75底盘程序，20ms一次/BSW_Output/CAN1_Tx/Subsystem/to28A/APA_28A1/APA_OnOff ==
  APA_OnOff : Inport
  APA_OnOffRon : Rounding  Operator=round
  APA_OnOff_1sat : Saturate  UpperLimit=64  LowerLimit=0
  APA_OnOff_Convert : DataTypeConversion  OutDataTypeStr=uint8
  APA_OnOff_Convert1 : DataTypeConversion  OutDataTypeStr=uint32
  APA_OnOff_D : Product  Inputs=*/
  APA_OnOff_F : Constant  OutDataTypeStr=single
  APA_OnOff_L : simulink/Logic and Bit Operations/Bitwise Operator  logicop=AND  UseBitMask=on  BitMask=64  BitMaskRealWorld=Stored Integer
  APA_OnOff_O : Constant  Value=0  OutDataTypeStr=single
  APA_OnOff_S : ArithShift  BitShiftNumber=-6
  APA_OnOff_sat : Saturate  UpperLimit=1  LowerLimit=0
  APA_OnOff_st : Sum  Inputs=+-
  Constant{2..8} (7 alike) : Constant  Value=0  OutDataTypeStr=uint8
  output1 : Outport
  output2 : Outport  Port=2
  output3 : Outport  Port=3
  output4 : Outport  Port=4
  output5 : Outport  Port=5
  output6 : Outport  Port=6
  output7 : Outport  Port=7
  output8 : Outport  Port=8
  wires:
  APA_OnOff/1 -> APA_OnOff_sat/1
  APA_OnOff_sat/1 -> APA_OnOff_st/1
  APA_OnOff_O/1 -> APA_OnOff_st/2
  APA_OnOff_st/1 -> APA_OnOff_D/1
  APA_OnOff_F/1 -> APA_OnOff_D/2
  APA_OnOff_D/1 -> APA_OnOffRon/1
  APA_OnOffRon/1 -> APA_OnOff_S/1
  APA_OnOff_S/1 -> APA_OnOff_1sat/1
  APA_OnOff_1sat/1 -> APA_OnOff_Convert1/1
  APA_OnOff_Convert1/1 -> APA_OnOff_L/1
  APA_OnOff_L/1 -> APA_OnOff_Convert/1
  APA_OnOff_Convert/1 -> output1/1
  Constant2/1 -> output2/1
  Constant3/1 -> output3/1
  Constant4/1 -> output4/1
  Constant5/1 -> output5/1
  Constant6/1 -> output6/1
  Constant7/1 -> output7/1
  Constant8/1 -> output8/1

== system VCU_CS75_9_30/长安CS75底盘程序，20ms一次/BSW_Output/CAN1_Tx/Subsystem/to28A/APA_28A1/APA_RollingCounter ==
  APA_RollingCounter : Inport
  APA_RollingCounterRon : Rounding  Operator=round
  APA_RollingCounter_1sat : Saturate  UpperLimit=15  LowerLimit=0
  APA_RollingCounter_Convert : DataTypeConversion  OutDataTypeStr=uint8
  APA_RollingCounter_Convert1 : DataTypeConversion  OutDataTypeStr=uint32
  APA_RollingCounter_D : Product  Inputs=*/
  APA_RollingCounter_F : Constant  OutDataTypeStr=single
  APA_RollingCounter_L : simulink/Logic and Bit Operations/Bitwise Operator  logicop=AND  UseBitMask=on  BitMask=15  BitMaskRealWorld=Stored Integer
  APA_RollingCounter_O : Constant  Value=0  OutDataTypeStr=single
  APA_RollingCounter_S : ArithShift
  APA_RollingCounter_sat : Saturate  UpperLimit=15  LowerLimit=0
  APA_RollingCounter_st : Sum  Inputs=+-
  Constant{1..6,8} (7 alike) : Constant  Value=0  OutDataTypeStr=uint8
  output1 : Outport
  output2 : Outport  Port=2
  output3 : Outport  Port=3
  output4 : Outport  Port=4
  output5 : Outport  Port=5
  output6 : Outport  Port=6
  output7 : Outport  Port=7
  output8 : Outport  Port=8
  wires:
  APA_RollingCounter/1 -> APA_RollingCounter_sat/1
  APA_RollingCounter_sat/1 -> APA_RollingCounter_st/1
  APA_RollingCounter_O/1 -> APA_RollingCounter_st/2
  APA_RollingCounter_st/1 -> APA_RollingCounter_D/1
  APA_RollingCounter_F/1 -> APA_RollingCounter_D/2
  APA_RollingCounter_D/1 -> APA_RollingCounterRon/1
  APA_RollingCounterRon/1 -> APA_RollingCounter_S/1
  APA_RollingCounter_S/1 -> APA_RollingCounter_1sat/1
  APA_RollingCounter_1sat/1 -> APA_RollingCounter_Convert1/1
  APA_RollingCounter_Convert1/1 -> APA_RollingCounter_L/1
  APA_RollingCounter_L/1 -> APA_RollingCounter_Convert/1
  APA_RollingCounter_Convert/1 -> output7/1
  Constant1/1 -> output1/1
  Constant2/1 -> output2/1
  Constant3/1 -> output3/1
  Constant4/1 -> output4/1
  Constant5/1 -> output5/1
  Constant6/1 -> output6/1
  Constant8/1 -> output8/1

== system VCU_CS75_9_30/长安CS75底盘程序，20ms一次/BSW_Output/CAN1_Tx/Subsystem/to28A/APA_28A1/APA_SteeringAngleReqProtection ==
  APA_SteeringAngleReqProtection : Inport
  APA_SteeringAngleReqProtectionRon : Rounding  Operator=round
  APA_SteeringAngleReqProtection_1sat : Saturate  UpperLimit=3  LowerLimit=0
  APA_SteeringAngleReqProtection_Convert : DataTypeConversion  OutDataTypeStr=uint8
  APA_SteeringAngleReqProtection_Convert1 : DataTypeConversion  OutDataTypeStr=uint32
  APA_SteeringAngleReqProtection_D : Product  Inputs=*/
  APA_SteeringAngleReqProtection_F : Constant  OutDataTypeStr=single
  APA_SteeringAngleReqProtection_L : simulink/Logic and Bit Operations/Bitwise Operator  logicop=AND  UseBitMask=on  BitMask=3  BitMaskRealWorld=Stored Integer
  APA_SteeringAngleReqProtection_O : Constant  Value=0  OutDataTypeStr=single
  APA_SteeringAngleReqProtection_S : ArithShift
  APA_SteeringAngleReqProtection_sat : Saturate  UpperLimit=3  LowerLimit=0
  APA_SteeringAngleReqProtection_st : Sum  Inputs=+-
  Constant{1..4,6..8} (7 alike) : Constant  Value=0  OutDataTypeStr=uint8
  output1 : Outport
  output2 : Outport  Port=2
  output3 : Outport  Port=3
  output4 : Outport  Port=4
  output5 : Outport  Port=5
  output6 : Outport  Port=6
  output7 : Outport  Port=7
  output8 : Outport  Port=8
  wires:
  APA_SteeringAngleReqProtection/1 -> APA_SteeringAngleReqProtection_sat/1
  APA_SteeringAngleReqProtection_sat/1 -> APA_SteeringAngleReqProtection_st/1
  APA_SteeringAngleReqProtection_O/1 -> APA_SteeringAngleReqProtection_st/2
  APA_SteeringAngleReqProtection_st/1 -> APA_SteeringAngleReqProtection_D/1
  APA_SteeringAngleReqProtection_F/1 -> APA_SteeringAngleReqProtection_D/2
  APA_SteeringAngleReqProtection_D/1 -> APA_SteeringAngleReqProtectionRon/1
  APA_SteeringAngleReqProtectionRon/1 -> APA_SteeringAngleReqProtection_S/1
  APA_SteeringAngleReqProtection_S/1 -> APA_SteeringAngleReqProtection_1sat/1
  APA_SteeringAngleReqProtection_1sat/1 -> APA_SteeringAngleReqProtection_Convert1/1
  APA_SteeringAngleReqProtection_Convert1/1 -> APA_SteeringAngleReqProtection_L/1
  APA_SteeringAngleReqProtection_L/1 -> APA_SteeringAngleReqProtection_Convert/1
  APA_SteeringAngleReqProtection_Convert/1 -> output5/1
  Constant1/1 -> output1/1
  Constant2/1 -> output2/1
  Constant3/1 -> output3/1
  Constant4/1 -> output4/1
  Constant6/1 -> output6/1
  Constant7/1 -> output7/1
  Constant8/1 -> output8/1

== system VCU_CS75_9_30/长安CS75底盘程序，20ms一次/BSW_Input/CAN0_Rx/a1_211/ReceiveMessages/Subsystem/a1/SCS_Sub ==
  In1 : Inport
  Out1 : Outport
  wires:
  In1/1 -> Out1/1

== system VCU_CS75_9_30/长安CS75底盘程序，20ms一次/BSW_Input/CAN0_Rx/a1_211/ReceiveMessages/Subsystem/a1/Vx_Sub ==
  In1 : Inport
  Out1 : Outport
  wires:
  In1/1 -> Out1/1

== system VCU_CS75_9_30/长安CS75底盘程序，20ms一次/BSW_Input/CAN0_Rx/a1_211/ReceiveMessages/Subsystem/a1/cones_count_actual_Sub ==
  In1 : Inport
  Out1 : Outport
  wires:
  In1/1 -> Out1/1

== system VCU_CS75_9_30/长安CS75底盘程序，20ms一次/BSW_Input/CAN0_Rx/a1_211/ReceiveMessages/Subsystem/a1/cones_count_all_Sub ==
  In1 : Inport
  Out1 : Outport
  wires:
  In1/1 -> Out1/1

== system VCU_CS75_9_30/长安CS75底盘程序，20ms一次/BSW_Input/CAN0_Rx/a1_211/ReceiveMessages/Subsystem/a1/finish_Sub ==
  In1 : Inport
  Out1 : Outport
  wires:
  In1/1 -> Out1/1

== system VCU_CS75_9_30/长安CS75底盘程序，20ms一次/BSW_Input/CAN0_Rx/a1_211/ReceiveMessages/Subsystem/a1/mission_Sub ==
  In1 : Inport
  Out1 : Outport
  wires:
  In1/1 -> Out1/1

== system VCU_CS75_9_30/长安CS75底盘程序，20ms一次/BSW_Input/CAN0_Rx/a1_211/ReceiveMessages/Subsystem/a1/tap_Sub ==
  In1 : Inport
  Out1 : Outport
  wires:
  In1/1 -> Out1/1

== system VCU_CS75_9_30/长安CS75底盘程序，20ms一次/BSW_Input/CAN0_Rx/a1_211/ReceiveMessages/Subsystem/a1/target_steering_Sub ==
  In1 : Inport
  Out1 : Outport
  wires:
  In1/1 -> Out1/1

== system VCU_CS75_9_30/长安CS75底盘程序，20ms一次/BSW_Input/CAN0_Rx/a1_211/ReceiveMessages/Subsystem/a1/throttlevbrake_position_Sub ==
  In1 : Inport
  Out1 : Outport
  wires:
  In1/1 -> Out1/1

== system VCU_CS75_9_30/长安CS75底盘程序，20ms一次/BSW_Input/CAN1_Rx/BCM_288/ReceiveMessages/Subsystem/BCM_1/BCM_BuzzerWarningMode_Sub ==
  In1 : Inport
  Out1 : Outport
  wires:
  In1/1 -> Out1/1

== system VCU_CS75_9_30/长安CS75底盘程序，20ms一次/BSW_Input/CAN1_Rx/BCM_288/ReceiveMessages/Subsystem/BCM_1/BCM_DriverDoorLockStatus_Sub ==
  In1 : Inport
  Out1 : Outport
  wires:
  In1/1 -> Out1/1

== system VCU_CS75_9_30/长安CS75底盘程序，20ms一次/BSW_Input/CAN1_Rx/BCM_288/ReceiveMessages/Subsystem/BCM_1/BCM_DriverDoorStatus_Sub ==
  In1 : Inport
  Out1 : Outport
  wires:
  In1/1 -> Out1/1

== system VCU_CS75_9_30/长安CS75底盘程序，20ms一次/BSW_Input/CAN1_Rx/BCM_288/ReceiveMessages/Subsystem/BCM_1/BCM_FrontWashStatus_Sub ==
  In1 : Inport
  Out1 : Outport
  wires:
  In1/1 -> Out1/1

== system VCU_CS75_9_30/长安CS75底盘程序，20ms一次/BSW_Input/CAN1_Rx/BCM_288/ReceiveMessages/Subsystem/BCM_1/BCM_FrontWiperStatus_Sub ==
  In1 : Inport
  Out1 : Outport
  wires:
  In1/1 -> Out1/1

== system VCU_CS75_9_30/长安CS75底盘程序，20ms一次/BSW_Input/CAN1_Rx/BCM_288/ReceiveMessages/Subsystem/BCM_1/BCM_HoodStatus_Sub ==
  In1 : Inport
  Out1 : Outport
  wires:
  In1/1 -> Out1/1

== system VCU_CS75_9_30/长安CS75底盘程序，20ms一次/BSW_Input/CAN1_Rx/BCM_288/ReceiveMessages/Subsystem/BCM_1/BCM_LatchOverheatProtect_Sub ==
  In1 : Inport
  Out1 : Outport
  wires:
  In1/1 -> Out1/1

== system VCU_CS75_9_30/长安CS75底盘程序，20ms一次/BSW_Input/CAN1_Rx/BCM_288/ReceiveMessages/Subsystem/BCM_1/BCM_LeftRearDoorStatus_Sub ==
  In1 : Inport
  Out1 : Outport
  wires:
  In1/1 -> Out1/1

== system VCU_CS75_9_30/长安CS75底盘程序，20ms一次/BSW_Input/CAN1_Rx/BCM_288/ReceiveMessages/Subsystem/BCM_1/BCM_PassengerDoorLockStatus_Sub ==
  In1 : Inport
  Out1 : Outport
  wires:
  In1/1 -> Out1/1

== system VCU_CS75_9_30/长安CS75底盘程序，20ms一次/BSW_Input/CAN1_Rx/BCM_288/ReceiveMessages/Subsystem/BCM_1/BCM_PassengerDoorStatus_Sub ==
  In1 : Inport
  Out1 : Outport
  wires:
  In1/1 -> Out1/1

== system VCU_CS75_9_30/长安CS75底盘程序，20ms一次/BSW_Input/CAN1_Rx/BCM_288/ReceiveMessages/Subsystem/BCM_1/BCM_PowerStatusFeedback_Sub ==
  In1 : Inport
  Out1 : Outport
  wires:
  In1/1 -> Out1/1

== system VCU_CS75_9_30/长安CS75底盘程序，20ms一次/BSW_Input/CAN1_Rx/BCM_288/ReceiveMessages/Subsystem/BCM_1/BCM_RearWiperStatus_Sub ==
  In1 : Inport
  Out1 : Outport
  wires:
  In1/1 -> Out1/1

== system VCU_CS75_9_30/长安CS75底盘程序，20ms一次/BSW_Input/CAN1_Rx/BCM_288/ReceiveMessages/Subsystem/BCM_1/BCM_ReversePosition_Sub ==
  In1 : Inport
  Out1 : Outport
  wires:
  In1/1 -> Out1/1

== system VCU_CS75_9_30/长安CS75底盘程序，20ms一次/BSW_Input/CAN1_Rx/BCM_288/ReceiveMessages/Subsystem/BCM_1/BCM_RightRearDoorStatus_Sub ==
  In1 : Inport
  Out1 : Outport
  wires:
  In1/1 -> Out1/1

== system VCU_CS75_9_30/长安CS75底盘程序，20ms一次/BSW_Input/CAN1_Rx/BCM_288/ReceiveMessages/Subsystem/BCM_1/BCM_SystemFailureFlag_Sub ==
  In1 : Inport
  Out1 : Outport
  wires:
  In1/1 -> Out1/1

== system VCU_CS75_9_30/长安CS75底盘程序，20ms一次/BSW_Input/CAN1_Rx/BCM_288/ReceiveMessages/Subsystem/BCM_1/BCM_TrunkDoorStatus_Sub ==
  In1 : Inport
  Out1 : Outport
  wires:
  In1/1 -> Out1/1

== system VCU_CS75_9_30/长安CS75底盘程序，20ms一次/BSW_Input/CAN1_Rx/BCM_288/ReceiveMessages/Subsystem/BCM_1/BCM_TurnIndicatorLeft_Sub ==
  In1 : Inport
  Out1 : Outport
  wires:
  In1/1 -> Out1/1

== system VCU_CS75_9_30/长安CS75底盘程序，20ms一次/BSW_Input/CAN1_Rx/BCM_288/ReceiveMessages/Subsystem/BCM_1/BCM_TurnIndicatorRight_Sub ==
  In1 : Inport
  Out1 : Outport
  wires:
  In1/1 -> Out1/1

== system VCU_CS75_9_30/长安CS75底盘程序，20ms一次/BSW_Input/CAN1_Rx/BCM_288/ReceiveMessages/Subsystem/BCM_1/BCM_TurnLightSwitchSts_Sub ==
  In1 : Inport
  Out1 : Outport
  wires:
  In1/1 -> Out1/1

== system VCU_CS75_9_30/长安CS75底盘程序，20ms一次/BSW_Input/CAN1_Rx/BCM_288/ReceiveMessages/Subsystem/BCM_1/BCM_emergencylightstatus_Sub ==
  In1 : Inport
  Out1 : Outport
  wires:
  In1/1 -> Out1/1

== system VCU_CS75_9_30/长安CS75底盘程序，20ms一次/BSW_Input/CAN1_Rx/BCM_328/ReceiveMessages/Subsystem/BCM_1/LCM_DRLSts_Sub ==
  In1 : Inport
  Out1 : Outport
  wires:
  In1/1 -> Out1/1

== system VCU_CS75_9_30/长安CS75底盘程序，20ms一次/BSW_Input/CAN1_Rx/BCM_328/ReceiveMessages/Subsystem/BCM_1/LCM_DriveMode_Sub ==
  In1 : Inport
  Out1 : Outport
  wires:
  In1/1 -> Out1/1

== system VCU_CS75_9_30/长安CS75底盘程序，20ms一次/BSW_Input/CAN1_Rx/BCM_328/ReceiveMessages/Subsystem/BCM_1/LCM_LASSwitch_Sub ==
  In1 : Inport
  Out1 : Outport
  wires:
  In1/1 -> Out1/1

== system VCU_CS75_9_30/长安CS75底盘程序，20ms一次/BSW_Input/CAN1_Rx/BCM_328/ReceiveMessages/Subsystem/BCM_1/LCM_RearLeftTuningLightFaultSts_Sub ==
  In1 : Inport
  Out1 : Outport
  wires:
  In1/1 -> Out1/1

== system VCU_CS75_9_30/长安CS75底盘程序，20ms一次/BSW_Input/CAN1_Rx/BCM_328/ReceiveMessages/Subsystem/BCM_1/LCM_RearRightTuningLightFaultSts_Sub ==
  In1 : Inport
  Out1 : Outport
  wires:
  In1/1 -> Out1/1

== system VCU_CS75_9_30/长安CS75底盘程序，20ms一次/BSW_Input/CAN1_Rx/BCM_328/ReceiveMessages/Subsystem/BCM_1/LCM_ReverseLightSts_Sub ==
  In1 : Inport
  Out1 : Outport
  wires:
  In1/1 -> Out1/1

== system VCU_CS75_9_30/长安CS75底盘程序，20ms一次/BSW_Input/CAN1_Rx/BCM_348/ReceiveMessages/Subsystem/BCM_1/BCM_DriveMode_Sub ==
  In1 : Inport
  Out1 : Outport
  wires:
  In1/1 -> Out1/1

== system VCU_CS75_9_30/长安CS75底盘程序，20ms一次/BSW_Input/CAN1_Rx/BCM_348/ReceiveMessages/Subsystem/BCM_1/BCM_LockSignal_Sub ==
  In1 : Inport
  Out1 : Outport
  wires:
  In1/1 -> Out1/1

== system VCU_CS75_9_30/长安CS75底盘程序，20ms一次/BSW_Input/CAN1_Rx/BCM_348/ReceiveMessages/Subsystem/BCM_1/BCM_UnlockSignal_Sub ==
  In1 : Inport
  Out1 : Outport
  wires:
  In1/1 -> Out1/1

== system VCU_CS75_9_30/长安CS75底盘程序，20ms一次/BSW_Input/CAN1_Rx/BCM_3DF/ReceiveMessages/Subsystem/BCM_3DF1/BCM_AmbientLightColorFeedback_Sub ==
  In1 : Inport
  Out1 : Outport
  wires:
  In1/1 -> Out1/1

== system VCU_CS75_9_30/长安CS75底盘程序，20ms一次/BSW_Input/CAN1_Rx/BCM_3DF/ReceiveMessages/Subsystem/BCM_3DF1/BCM_CRC_Checksum_Sub ==
  In1 : Inport
  Out1 : Outport
  wires:
  In1/1 -> Out1/1

== system VCU_CS75_9_30/长安CS75底盘程序，20ms一次/BSW_Input/CAN1_Rx/BCM_3DF/ReceiveMessages/Subsystem/BCM_3DF1/BCM_DriveModeFeedback_Sub ==
  In1 : Inport
  Out1 : Outport
  wires:
  In1/1 -> Out1/1

== system VCU_CS75_9_30/长安CS75底盘程序，20ms一次/BSW_Input/CAN1_Rx/BCM_3DF/ReceiveMessages/Subsystem/BCM_3DF1/BCM_DriveModeStatus_Sub ==
  In1 : Inport
  Out1 : Outport
  wires:
  In1/1 -> Out1/1

== system VCU_CS75_9_30/长安CS75底盘程序，20ms一次/BSW_Input/CAN1_Rx/BCM_3DF/ReceiveMessages/Subsystem/BCM_3DF1/BCM_DriveMode_Sub ==
  In1 : Inport
  Out1 : Outport
  wires:
  In1/1 -> Out1/1

== system VCU_CS75_9_30/长安CS75底盘程序，20ms一次/BSW_Input/CAN1_Rx/BCM_3DF/ReceiveMessages/Subsystem/BCM_3DF1/BCM_EPSTorqueModeFeedback_Sub ==
  In1 : Inport
  Out1 : Outport
  wires:
  In1/1 -> Out1/1

== system VCU_CS75_9_30/长安CS75底盘程序，20ms一次/BSW_Input/CAN1_Rx/BCM_3DF/ReceiveMessages/Subsystem/BCM_3DF1/BCM_EPSTorqueMode_Sub ==
  In1 : Inport
  Out1 : Outport
  wires:
  In1/1 -> Out1/1

== system VCU_CS75_9_30/长安CS75底盘程序，20ms一次/BSW_Input/CAN1_Rx/BCM_3DF/ReceiveMessages/Subsystem/BCM_3DF1/BCM_RollingCounter_Sub ==
  In1 : Inport
  Out1 : Outport
  wires:
  In1/1 -> Out1/1

== system VCU_CS75_9_30/长安CS75底盘程序，20ms一次/BSW_Input/CAN1_Rx/EMS_205/ReceiveMessages/Subsystem/EMS/EMS_CheckSum_205_Sub ==
  In1 : Inport
  Out1 : Outport
  wires:
  In1/1 -> Out1/1

== system VCU_CS75_9_30/长安CS75底盘程序，20ms一次/BSW_Input/CAN1_Rx/EMS_205/ReceiveMessages/Subsystem/EMS/EMS_ESPTorqReuestAvailability_Sub ==
  In1 : Inport
  Out1 : Outport
  wires:
  In1/1 -> Out1/1

== system VCU_CS75_9_30/长安CS75底盘程序，20ms一次/BSW_Input/CAN1_Rx/EMS_205/ReceiveMessages/Subsystem/EMS/EMS_FrictionalTorq_Sub ==
  In1 : Inport
  Out1 : Outport
  wires:
  In1/1 -> Out1/1

== system VCU_CS75_9_30/长安CS75底盘程序，20ms一次/BSW_Input/CAN1_Rx/EMS_205/ReceiveMessages/Subsystem/EMS/EMS_IndicatedDriverReqTorq_Sub ==
  In1 : Inport
  Out1 : Outport
  wires:
  In1/1 -> Out1/1

== system VCU_CS75_9_30/长安CS75底盘程序，20ms一次/BSW_Input/CAN1_Rx/EMS_205/ReceiveMessages/Subsystem/EMS/EMS_IndicatedRealEngTorq_Sub ==
  In1 : Inport
  Out1 : Outport
  wires:
  In1/1 -> Out1/1

== system VCU_CS75_9_30/长安CS75底盘程序，20ms一次/BSW_Input/CAN1_Rx/EMS_205/ReceiveMessages/Subsystem/EMS/EMS_RollingCounter_id205_Sub ==
  In1 : Inport
  Out1 : Outport
  wires:
  In1/1 -> Out1/1

== system VCU_CS75_9_30/长安CS75底盘程序，20ms一次/BSW_Input/CAN1_Rx/EMS_205/ReceiveMessages/Subsystem/EMS/EMS_TorqFailure_Sub ==
  In1 : Inport
  Out1 : Outport
  wires:
  In1/1 -> Out1/1

== system VCU_CS75_9_30/长安CS75底盘程序，20ms一次/BSW_Input/CAN1_Rx/EMS_255/ReceiveMessages/Subsystem/EMS/EMS_AccPedal_Sub ==
  In1 : Inport
  Out1 : Outport
  wires:
  In1/1 -> Out1/1

== system VCU_CS75_9_30/长安CS75底盘程序，20ms一次/BSW_Input/CAN1_Rx/EMS_255/ReceiveMessages/Subsystem/EMS/EMS_AccpedelError_Sub ==
  In1 : Inport
  Out1 : Outport
  wires:
  In1/1 -> Out1/1

== system VCU_CS75_9_30/长安CS75底盘程序，20ms一次/BSW_Input/CAN1_Rx/EMS_255/ReceiveMessages/Subsystem/EMS/EMS_BrakePedalStatus_Sub ==
  In1 : Inport
  Out1 : Outport
  wires:
  In1/1 -> Out1/1

== system VCU_CS75_9_30/长安CS75底盘程序，20ms一次/BSW_Input/CAN1_Rx/EMS_255/ReceiveMessages/Subsystem/EMS/EMS_CheckSum_255_Sub ==
  In1 : Inport
  Out1 : Outport
  wires:
  In1/1 -> Out1/1

== system VCU_CS75_9_30/长安CS75底盘程序，20ms一次/BSW_Input/CAN1_Rx/EMS_255/ReceiveMessages/Subsystem/EMS/EMS_EngineSpeedError_Sub ==
  In1 : Inport
  Out1 : Outport
  wires:
  In1/1 -> Out1/1

== system VCU_CS75_9_30/长安CS75底盘程序，20ms一次/BSW_Input/CAN1_Rx/EMS_255/ReceiveMessages/Subsystem/EMS/EMS_EngineSpeed_Sub ==
  In1 : Inport
  Out1 : Outport
  wires:
  In1/1 -> Out1/1

== system VCU_CS75_9_30/长安CS75底盘程序，20ms一次/BSW_Input/CAN1_Rx/EMS_255/ReceiveMessages/Subsystem/EMS/EMS_RollingCounter_id255_Sub ==
  In1 : Inport
  Out1 : Outport
  wires:
  In1/1 -> Out1/1

== system VCU_CS75_9_30/长安CS75底盘程序，20ms一次/BSW_Input/CAN1_Rx/EMS_265/ReceiveMessages/Subsystem/EMS_265xx/EMS_EngineStatus_Sub ==
  In1 : Inport
  Out1 : Outport
  wires:
  In1/1 -> Out1/1

== system VCU_CS75_9_30/长安CS75底盘程序，20ms一次/BSW_Input/CAN1_Rx/EMS_265/ReceiveMessages/Subsystem/EMS_265xx/EMS_FullLoadIndicatedTorq_Sub ==
  In1 : Inport
  Out1 : Outport
  wires:
  In1/1 -> Out1/1
